simulink model "ACStesbed"  (R2015b)
settings: Solver=ode45  StartTime=0.0  StopTime=1500  FixedStep=0.02  RelTol=1e-3
StartFcn:
  | InitializeModel
values from neighbouring files (symbols this model uses):
  D = L+eye(3)    [controllability.m]    (also in func.m = skewsym(X(2:4))+eye(3); func1.m = skewsym(X(2:4))+eye(3); kab2.m = Dt'; sys1.m = skewsym(X0(2:4))+eye(3))
undefined symbols (not defined in the file or in its folder): DiscIntNeverNeededParam, e0_0, e1_0, e2_0, e3_0, OrbData, params
libraries: aerolibutil x16, vrlib x13, satellite_control_lib x8, dspmtrx3 x4, aerolibtransform2 x3, aerolib6dofsys x2, simulink x2, aerolib6dof2 x1, dspinverses x1, dspmathops x1
(part 2 of 2)

== matlab function ACStesbed/TestBedComputer/VerEst/Unscented Kalman Filter ==
  data: W input; rz_estin input; W_estin input; Pin input; rz_est output; dh input; h input; gb input; J input; W_est output; P output; Mass input
function [ rz_est,W_est,P ] = VertUKF(W,rz_estin,W_estin,Pin,dh,h,gb,J,Mass)
%VertUKF Оценка вертикальной составляющей смещения центра масс с помощью
%сигма-точечного фильтра Калмана
x=[W_estin; rz_estin];
q=1e-6;										%std of process 
r=5e-6;										%std of measurement
Q=[q^2*eye(3),zeros(3,1);zeros(1,3),(1e-6)^2];									% covariance of process
R=r^2*eye(3);										% covariance of measurement 
[x,P]=ukf(@F,x,Pin,@H,W,Q,R,dh,h,gb,J,Mass);
W_est=x(1:3);
rz_est=x(4);
end

% nonlinear state equations
function [Y] = F(x,dh,h,gb,J,Mass)
Y=x+0.1*[J^-1*(-cross(x(1:3),J*x(1:3)+h)-dh+Mass*x(4)*[-gb(2);gb(1);0]);0];
end
% function of measurments
function [Z] = H(x,dh,h,gb,J,Mass)
Z=[x(1);x(2);x(3)];
end

function [x,P]=ukf(fstate,x,P,hmeas,z,Q,R,dh,h,gb,J,Mass)
% UKF   Unscented Kalman Filter for nonlinear dynamic systems
% [x, P] = ukf(f,x,P,h,z,Q,R) returns state estimate, x and state covariance, P 
% for nonlinear dynamic system (for simplicity, noises are assumed as additive):
%           x_k+1 = f(x_k) + w_k
%           z_k   = h(x_k) + v_k
% where w ~ N(0,Q) meaning w is gaussian noise with covariance Q
%       v ~ N(0,R) meaning v is gaussian noise with covariance R
% Inputs:   f: function handle for f(x)
%           x: "a priori" state estimate
%           P: "a priori" estimated state covariance
%           h: fanction handle for h(x)
%           z: current measurement
%           Q: process noise covariance 
%           R: measurement noise covariance
% Output:   x: "a posteriori" state estimate
%           P: "a posteriori" state covariance
%
% Example:
%{
n=3;      %number of state
q=0.1;    %std of process 
r=0.1;    %std of measurement
Q=q^2*eye(n); % covariance of process
R=r^2;        % covariance of measurement  
f=@(x)[x(2);x(3);0.05*x(1)*(x(2)+x(3))];  % nonlinear state equations
h=@(x)x(1);                               % measurement equation
s=[0;0;1];                                % initial state
x=s+q*randn(3,1); %initial state          % initial state with noise
P = eye(n);                               % initial state covraiance
N=20;                                     % total dynamic steps
xV = zeros(n,N);          %estmate        % allocate memory
sV = zeros(n,N);          %actual
zV = zeros(1,N);
for k=1:N
  z = h(s) + r*randn;                     % measurments
  sV(:,k)= s;                             % save actual state
  zV(k)  = z;                             % save measurment
  [x, P] = ukf(f,x,P,h,z,Q,R);            % ekf 
  xV(:,k) = x;                            % save estimate
  s = f(s) + q*randn(3,1);                % update process 
end
for k=1:3                                 % plot results
  subplot(3,1,k)
  plot(1:N, sV(k,:), '-', 1:N, xV(k,:), '--')
end
%}
% Reference: Julier, SJ. and Uhlmann, J.K., Unscented Filtering and
% Nonlinear Estimation, Proceedings of the IEEE, Vol. 92, No. 3,
% pp.401-422, 2004. 
%
% By Yi Cao at Cranfield University, 04/01/2008
%
L=numel(x);                                 %numer of states
m=numel(z);                                 %numer of measurements
alpha=1e-3;                                 %default, tunable
ki=0;                                       %default, tunable
beta=2;                                     %default, tunable
lambda=alpha^2*(L+ki)-L;                    %scaling factor
c=L+lambda;                                 %scaling factor
Wm=[lambda/c 0.5/c+zeros(1,2*L)];           %weights for means
Wc=Wm;
Wc(1)=Wc(1)+(1-alpha^2+beta);               %weights for covariance
c=sqrt(c);
X=sigmas(x,P,c);                            %sigma points around x
[x1,X1,P1,X2]=ut(fstate,X,Wm,Wc,L,Q,dh,h,gb,J,Mass);          %unscented transformation of process
% X1=sigmas(x1,P1,c);                         %sigma points around x1
% X2=X1-x1(:,ones(1,size(X1,2)));             %deviation of X1
[z1,Z1,P2,Z2]=ut(hmeas,X1,Wm,Wc,m,R,dh,h,gb,J,Mass);       %unscented transformation of measurments
P12=X2*diag(Wc)*Z2';                        %transformed cross-covariance
K=P12*inv(P2);
x=x1+K*(z-z1);                              %state update
P=P1-K*P12';                                %covariance update
end

function [y,Y,P,Y1]=ut(func,X,Wm,Wc,n,R,dh,h,gb,J,Mass)
%Unscented Transformation
%Input:
%        f: nonlinear map
%        X: sigma points
%       Wm: weights for mean
%       Wc: weights for covariance
%        n: numer of outputs of f
%        R: additive covariance
%Output:
%        y: transformed mean
%        Y: transformed smapling points
%        P: transformed covariance
%       Y1: transformed deviations

L=size(X,2);
y=zeros(n,1);
Y=zeros(n,L);
for k=1:L                   
    Y(:,k)=func(X(:,k),dh,h,gb,J,Mass);       
    y=y+Wm(k)*Y(:,k);       
end
Y1=Y-y(:,ones(1,L));
P=Y1*diag(Wc)*Y1'+R; 
end

function X=sigmas(x,P,c)
%Sigma points around reference point
%Inputs:
%       x: reference point
%       P: covariance
%       c: coefficient
%Output:
%       X: Sigma points

A = c*chol(P)';
Y = x(:,ones(1,numel(x)));
X = [x Y+A Y-A]; 
end
